simulink library "DB42S03"  (R2024b)
settings: Solver=VariableStepAuto  StartTime=0.0  StopTime=10.0  RelTol=1e-3
libraries: autolibbldc x1
settings Model: Creator=folke  LastModifiedBy=folke

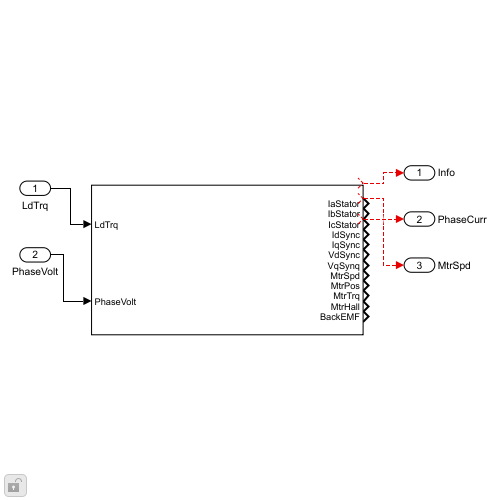
[thumbnail: Simulink's stored preview of the top-level diagram]
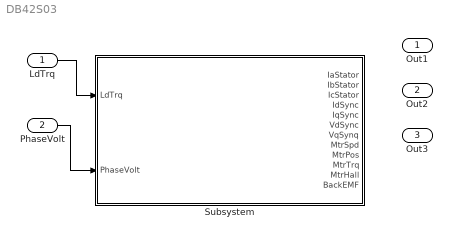
== system DB42S03 ==
  LdTrq : Inport
  PhaseVolt : Inport  Port=2
  Subsystem : Subsystem
  Out1 : Outport  SignalName=Info
  Out2 : Outport  Port=2  SignalName=PhaseCurr
  Out3 : Outport  Port=3  SignalName=MtrSpd
  wires:
  LdTrq/1 -> Subsystem/1(LdTrq)
  PhaseVolt/1 -> Subsystem/2(PhaseVolt)
  ? -> Out1/1
  ? -> Out2/1
  ? -> Out3/1

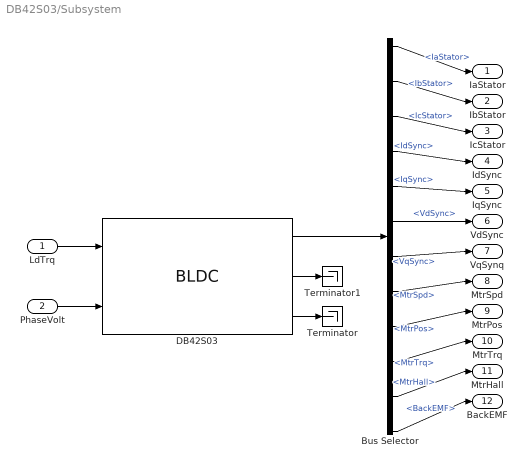
== system DB42S03/Subsystem ==
  LdTrq : Inport
  PhaseVolt : Inport  Port=2
  Bus Selector : BusSelector  OutputSignals=IaStator,IbStator,IcStator,IdSync,IqSync,VdSync,VqSync,MtrSpd,MtrPos,MtrTrq,MtrHall,BackEMF
  DB42S03 : autolibbldc/BLDC  VariantControl=pmsmVariant==pmsmEnum.TorqueInput  MechInput=Torque  SimType=Discrete  BlockSampleTime=10e-6  p=4  Rs=0.7  Ld=0.0006  Lq=0.0006  Lambda=0.00583  J=2.4e-06  B=2.6369e-06  F=0  Id_init=0  Iq_init=0  Th_init=0  Omega_init=0  RefBlkName='autolibbldc/BLDC'  aMode=5
      settings: LibrarySourceBlock=mcblib/Electrical Systems/Motors/BLDC
  Terminator : Terminator
  Terminator1 : Terminator
  IaStator : Outport
  IbStator : Outport  Port=2
  IcStator : Outport  Port=3
  IdSync : Outport  Port=4
  IqSync : Outport  Port=5
  VdSync : Outport  Port=6
  VqSynq : Outport  Port=7
  MtrSpd : Outport  Port=8
  MtrPos : Outport  Port=9
  MtrTrq : Outport  Port=10
  MtrHall : Outport  Port=11
  BackEMF : Outport  Port=12
  wires:
  LdTrq/1 -> DB42S03/1
  PhaseVolt/1 -> DB42S03/2
  DB42S03/1 -> Bus Selector/1
  Bus Selector/1 -> IaStator/1  "<IaStator>"
  Bus Selector/2 -> IbStator/1  "<IbStator>"
  Bus Selector/3 -> IcStator/1  "<IcStator>"
  Bus Selector/4 -> IdSync/1  "<IdSync>"
  Bus Selector/5 -> IqSync/1  "<IqSync>"
  Bus Selector/6 -> VdSync/1  "<VdSync>"
  Bus Selector/7 -> VqSynq/1  "<VqSync>"
  Bus Selector/8 -> MtrSpd/1  "<MtrSpd>"
  Bus Selector/9 -> MtrPos/1  "<MtrPos>"
  Bus Selector/10 -> MtrTrq/1  "<MtrTrq>"
  Bus Selector/11 -> MtrHall/1  "<MtrHall>"
  Bus Selector/12 -> BackEMF/1  "<BackEMF>"
  DB42S03/3 -> Terminator/1
  DB42S03/2 -> Terminator1/1
